simulink library "BFDAMP_MASTER"  (Simulink 8.5)
settings: Solver=ode45  StartTime=0.0  StopTime=10.0  RelTol=1e-3
libraries: cdsEpicsOut x36, cdsTP x18, cdsFiltCtrl x12, cdsFilt x12, cdsEpicsIn x7, cdsRms x6, cdsMuxMatrix x2, cdsEpicsBinIn x1, cdsFunctionCall x1, SIXOSEM_F_WD_AC_MASTER x1
(part 3 of 3)

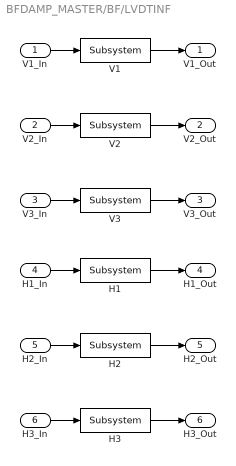
== system BFDAMP_MASTER/BF/LVDTINF ==
  V1_In : Inport
  V2_In : Inport  Port=2
  V3_In : Inport  Port=3
  H1_In : Inport  Port=4
  H2_In : Inport  Port=5
  H3_In : Inport  Port=6
  H1 : cdsFilt/Subsystem  Tag=cdsFilt  Description=|
      | Purpose:                                                                                                                                                                                                                                  
      | Standard CDS IIR filter module.                                                                                                                                                                                                           
      |                                                                                                                                                                                                                                           
      | Operation:                                                                                                                                                                                                                                
      | Consists of 10 second order section IIR filters, plus a ramped gain stage. In FE code, also provides pre-defined test points and excitation channel inputs. The filter coefficients are defined in the LIGO system using the 'foton' tool.
      |                                                                                                                                                                                                                                           
      | Usage:                                                                                                                                                                                                                                    
      | Name the part with the desired filter module name.
      settings: AttributesFormatString=%<Tag>
  H2 : cdsFilt/Subsystem  Tag=cdsFilt  Description=|
      | Purpose:                                                                                                                                                                                                                                  
      | Standard CDS IIR filter module.                                                                                                                                                                                                           
      |                                                                                                                                                                                                                                           
      | Operation:                                                                                                                                                                                                                                
      | Consists of 10 second order section IIR filters, plus a ramped gain stage. In FE code, also provides pre-defined test points and excitation channel inputs. The filter coefficients are defined in the LIGO system using the 'foton' tool.
      |                                                                                                                                                                                                                                           
      | Usage:                                                                                                                                                                                                                                    
      | Name the part with the desired filter module name.
      settings: AttributesFormatString=%<Tag>
  H3 : cdsFilt/Subsystem  Tag=cdsFilt  Description=|
      | Purpose:                                                                                                                                                                                                                                  
      | Standard CDS IIR filter module.                                                                                                                                                                                                           
      |                                                                                                                                                                                                                                           
      | Operation:                                                                                                                                                                                                                                
      | Consists of 10 second order section IIR filters, plus a ramped gain stage. In FE code, also provides pre-defined test points and excitation channel inputs. The filter coefficients are defined in the LIGO system using the 'foton' tool.
      |                                                                                                                                                                                                                                           
      | Usage:                                                                                                                                                                                                                                    
      | Name the part with the desired filter module name.
      settings: AttributesFormatString=%<Tag>
  V1 : cdsFilt/Subsystem  Tag=cdsFilt  Description=|
      | Purpose:                                                                                                                                                                                                                                  
      | Standard CDS IIR filter module.                                                                                                                                                                                                           
      |                                                                                                                                                                                                                                           
      | Operation:                                                                                                                                                                                                                                
      | Consists of 10 second order section IIR filters, plus a ramped gain stage. In FE code, also provides pre-defined test points and excitation channel inputs. The filter coefficients are defined in the LIGO system using the 'foton' tool.
      |                                                                                                                                                                                                                                           
      | Usage:                                                                                                                                                                                                                                    
      | Name the part with the desired filter module name.
      settings: AttributesFormatString=%<Tag>
  V2 : cdsFilt/Subsystem  Tag=cdsFilt  Description=|
      | Purpose:                                                                                                                                                                                                                                  
      | Standard CDS IIR filter module.                                                                                                                                                                                                           
      |                                                                                                                                                                                                                                           
      | Operation:                                                                                                                                                                                                                                
      | Consists of 10 second order section IIR filters, plus a ramped gain stage. In FE code, also provides pre-defined test points and excitation channel inputs. The filter coefficients are defined in the LIGO system using the 'foton' tool.
      |                                                                                                                                                                                                                                           
      | Usage:                                                                                                                                                                                                                                    
      | Name the part with the desired filter module name.
      settings: AttributesFormatString=%<Tag>
  V3 : cdsFilt/Subsystem  Tag=cdsFilt  Description=|
      | Purpose:                                                                                                                                                                                                                                  
      | Standard CDS IIR filter module.                                                                                                                                                                                                           
      |                                                                                                                                                                                                                                           
      | Operation:                                                                                                                                                                                                                                
      | Consists of 10 second order section IIR filters, plus a ramped gain stage. In FE code, also provides pre-defined test points and excitation channel inputs. The filter coefficients are defined in the LIGO system using the 'foton' tool.
      |                                                                                                                                                                                                                                           
      | Usage:                                                                                                                                                                                                                                    
      | Name the part with the desired filter module name.
      settings: AttributesFormatString=%<Tag>
  V1_Out : Outport
  V2_Out : Outport  Port=2
  V3_Out : Outport  Port=3
  H1_Out : Outport  Port=4
  H2_Out : Outport  Port=5
  H3_Out : Outport  Port=6
  wires:
  V1_In/1 -> V1/1
  V1/1 -> V1_Out/1
  V2_In/1 -> V2/1
  V2/1 -> V2_Out/1
  V3_In/1 -> V3/1
  V3/1 -> V3_Out/1
  H1_In/1 -> H1/1
  H1/1 -> H1_Out/1
  H2_In/1 -> H2/1
  H2/1 -> H2_Out/1
  H3_In/1 -> H3/1
  H3/1 -> H3_Out/1

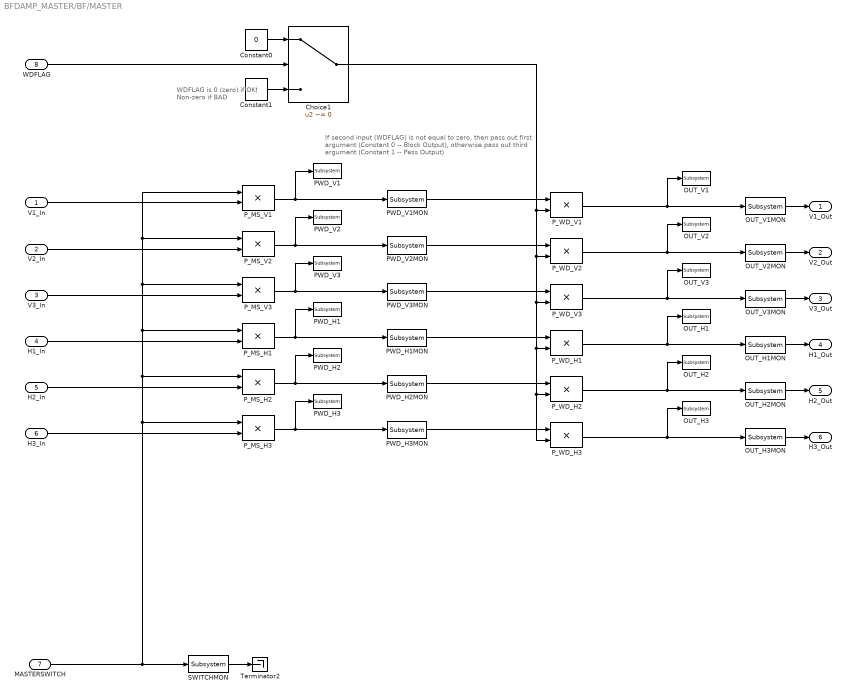
== system BFDAMP_MASTER/BF/MASTER ==
  note: If second input (WDFLAG) is not equal to zero,
      | then pass out first argument (Constant 0 -- Block Output),
      | otherwise pass out third argument (Constant 1 -- Pass Output)
  note: WDFLAG is 0 (zero) if OK,
      | Non-zero if BAD
  V1_In : Inport
  V2_In : Inport  Port=2
  V3_In : Inport  Port=3
  H1_In : Inport  Port=4
  H2_In : Inport  Port=5
  H3_In : Inport  Port=6
  MASTERSWITCH : Inport  Port=7
  WDFLAG : Inport  Port=8
  Choice1 : Switch  Criteria=u2 ~= 0  Threshold=0.5
  Constant0 : Constant  Value=0
  Constant1 : Constant
  OUT_H1 : cdsTP/Subsystem  Tag=Test Point
      settings: AttributesFormatString=%<Tag>
  OUT_H1MON : cdsEpicsOut/Subsystem  Tag=cdsEpicsOutput  Description=|
      | Purpose:                                          
      | Output a FE signal to an EPICS channel.           
      |                                                   
      | Operation:                                        
      | Takes input value and passes it to EPICS record.  
      |                                                   
      | Usage:                                            
      | Name the part with the desired EPICS rrecord name.
      settings: AttributesFormatString=%<Tag>
  OUT_H2 : cdsTP/Subsystem  Tag=Test Point
      settings: AttributesFormatString=%<Tag>
  OUT_H2MON : cdsEpicsOut/Subsystem  Tag=cdsEpicsOutput  Description=|
      | Purpose:                                          
      | Output a FE signal to an EPICS channel.           
      |                                                   
      | Operation:                                        
      | Takes input value and passes it to EPICS record.  
      |                                                   
      | Usage:                                            
      | Name the part with the desired EPICS rrecord name.
      settings: AttributesFormatString=%<Tag>
  OUT_H3 : cdsTP/Subsystem  Tag=Test Point
      settings: AttributesFormatString=%<Tag>
  OUT_H3MON : cdsEpicsOut/Subsystem  Tag=cdsEpicsOutput  Description=|
      | Purpose:                                          
      | Output a FE signal to an EPICS channel.           
      |                                                   
      | Operation:                                        
      | Takes input value and passes it to EPICS record.  
      |                                                   
      | Usage:                                            
      | Name the part with the desired EPICS rrecord name.
      settings: AttributesFormatString=%<Tag>
  OUT_V1 : cdsTP/Subsystem  Tag=Test Point
      settings: AttributesFormatString=%<Tag>
  OUT_V1MON : cdsEpicsOut/Subsystem  Tag=cdsEpicsOutput  Description=|
      | Purpose:                                          
      | Output a FE signal to an EPICS channel.           
      |                                                   
      | Operation:                                        
      | Takes input value and passes it to EPICS record.  
      |                                                   
      | Usage:                                            
      | Name the part with the desired EPICS rrecord name.
      settings: AttributesFormatString=%<Tag>
  OUT_V2 : cdsTP/Subsystem  Tag=Test Point
      settings: AttributesFormatString=%<Tag>
  OUT_V2MON : cdsEpicsOut/Subsystem  Tag=cdsEpicsOutput  Description=|
      | Purpose:                                          
      | Output a FE signal to an EPICS channel.           
      |                                                   
      | Operation:                                        
      | Takes input value and passes it to EPICS record.  
      |                                                   
      | Usage:                                            
      | Name the part with the desired EPICS rrecord name.
      settings: AttributesFormatString=%<Tag>
  OUT_V3 : cdsTP/Subsystem  Tag=Test Point
      settings: AttributesFormatString=%<Tag>
  OUT_V3MON : cdsEpicsOut/Subsystem  Tag=cdsEpicsOutput  Description=|
      | Purpose:                                          
      | Output a FE signal to an EPICS channel.           
      |                                                   
      | Operation:                                        
      | Takes input value and passes it to EPICS record.  
      |                                                   
      | Usage:                                            
      | Name the part with the desired EPICS rrecord name.
      settings: AttributesFormatString=%<Tag>
  PWD_H1 : cdsTP/Subsystem  Tag=Test Point
      settings: AttributesFormatString=%<Tag>
  PWD_H1MON : cdsEpicsOut/Subsystem  Tag=cdsEpicsOutput  Description=|
      | Purpose:                                          
      | Output a FE signal to an EPICS channel.           
      |                                                   
      | Operation:                                        
      | Takes input value and passes it to EPICS record.  
      |                                                   
      | Usage:                                            
      | Name the part with the desired EPICS rrecord name.
      settings: AttributesFormatString=%<Tag>
  PWD_H2 : cdsTP/Subsystem  Tag=Test Point
      settings: AttributesFormatString=%<Tag>
  PWD_H2MON : cdsEpicsOut/Subsystem  Tag=cdsEpicsOutput  Description=|
      | Purpose:                                          
      | Output a FE signal to an EPICS channel.           
      |                                                   
      | Operation:                                        
      | Takes input value and passes it to EPICS record.  
      |                                                   
      | Usage:                                            
      | Name the part with the desired EPICS rrecord name.
      settings: AttributesFormatString=%<Tag>
  PWD_H3 : cdsTP/Subsystem  Tag=Test Point
      settings: AttributesFormatString=%<Tag>
  PWD_H3MON : cdsEpicsOut/Subsystem  Tag=cdsEpicsOutput  Description=|
      | Purpose:                                          
      | Output a FE signal to an EPICS channel.           
      |                                                   
      | Operation:                                        
      | Takes input value and passes it to EPICS record.  
      |                                                   
      | Usage:                                            
      | Name the part with the desired EPICS rrecord name.
      settings: AttributesFormatString=%<Tag>
  PWD_V1 : cdsTP/Subsystem  Tag=Test Point
      settings: AttributesFormatString=%<Tag>
  PWD_V1MON : cdsEpicsOut/Subsystem  Tag=cdsEpicsOutput  Description=|
      | Purpose:                                          
      | Output a FE signal to an EPICS channel.           
      |                                                   
      | Operation:                                        
      | Takes input value and passes it to EPICS record.  
      |                                                   
      | Usage:                                            
      | Name the part with the desired EPICS rrecord name.
      settings: AttributesFormatString=%<Tag>
  PWD_V2 : cdsTP/Subsystem  Tag=Test Point
      settings: AttributesFormatString=%<Tag>
  PWD_V2MON : cdsEpicsOut/Subsystem  Tag=cdsEpicsOutput  Description=|
      | Purpose:                                          
      | Output a FE signal to an EPICS channel.           
      |                                                   
      | Operation:                                        
      | Takes input value and passes it to EPICS record.  
      |                                                   
      | Usage:                                            
      | Name the part with the desired EPICS rrecord name.
      settings: AttributesFormatString=%<Tag>
  PWD_V3 : cdsTP/Subsystem  Tag=Test Point
      settings: AttributesFormatString=%<Tag>
  PWD_V3MON : cdsEpicsOut/Subsystem  Tag=cdsEpicsOutput  Description=|
      | Purpose:                                          
      | Output a FE signal to an EPICS channel.           
      |                                                   
      | Operation:                                        
      | Takes input value and passes it to EPICS record.  
      |                                                   
      | Usage:                                            
      | Name the part with the desired EPICS rrecord name.
      settings: AttributesFormatString=%<Tag>
  P_MS_H1 : Product  RndMeth=Zero
  P_MS_H2 : Product  RndMeth=Zero
  P_MS_H3 : Product  RndMeth=Zero
  P_MS_V1 : Product  RndMeth=Zero
  P_MS_V2 : Product  RndMeth=Zero
  P_MS_V3 : Product  RndMeth=Zero
  P_WD_H1 : Product  RndMeth=Zero
  P_WD_H2 : Product  RndMeth=Zero
  P_WD_H3 : Product  RndMeth=Zero
  P_WD_V1 : Product  RndMeth=Zero
  P_WD_V2 : Product  RndMeth=Zero
  P_WD_V3 : Product  RndMeth=Zero
  SWITCHMON : cdsEpicsOut/Subsystem  Tag=cdsEpicsOutput  Description=|
      | Purpose:                                          
      | Output a FE signal to an EPICS channel.           
      |                                                   
      | Operation:                                        
      | Takes input value and passes it to EPICS record.  
      |                                                   
      | Usage:                                            
      | Name the part with the desired EPICS rrecord name.
      settings: AttributesFormatString=%<Tag>
  Terminator2 : Terminator
  V1_Out : Outport
  V2_Out : Outport  Port=2
  V3_Out : Outport  Port=3
  H1_Out : Outport  Port=4
  H2_Out : Outport  Port=5
  H3_Out : Outport  Port=6
  wires:
  SWITCHMON/1 -> Terminator2/1
  V1_In/1 -> P_MS_V1/2
  V2_In/1 -> P_MS_V2/2
  V3_In/1 -> P_MS_V3/2
  H1_In/1 -> P_MS_H1/2
  H2_In/1 -> P_MS_H2/2
  H3_In/1 -> P_MS_H3/2
  MASTERSWITCH/1 -> SWITCHMON/1, P_MS_V1/1, P_MS_V2/1, P_MS_V3/1, P_MS_H1/1, P_MS_H2/1, P_MS_H3/1
  OUT_V2MON/1 -> V2_Out/1
  OUT_V1MON/1 -> V1_Out/1
  OUT_V3MON/1 -> V3_Out/1
  OUT_H1MON/1 -> H1_Out/1
  OUT_H3MON/1 -> H3_Out/1
  OUT_H2MON/1 -> H2_Out/1
  P_MS_V1/1 -> PWD_V1/1, PWD_V1MON/1
  P_MS_V2/1 -> PWD_V2/1, PWD_V2MON/1
  P_MS_V3/1 -> PWD_V3/1, PWD_V3MON/1
  P_MS_H1/1 -> PWD_H1/1, PWD_H1MON/1
  P_MS_H2/1 -> PWD_H2/1, PWD_H2MON/1
  P_MS_H3/1 -> PWD_H3/1, PWD_H3MON/1
  P_WD_V1/1 -> OUT_V1MON/1, OUT_V1/1
  P_WD_V2/1 -> OUT_V2MON/1, OUT_V2/1
  P_WD_V3/1 -> OUT_V3MON/1, OUT_V3/1
  P_WD_H1/1 -> OUT_H1MON/1, OUT_H1/1
  P_WD_H2/1 -> OUT_H2MON/1, OUT_H2/1
  P_WD_H3/1 -> OUT_H3MON/1, OUT_H3/1
  Constant1/1 -> Choice1/3
  Constant0/1 -> Choice1/1
  WDFLAG/1 -> Choice1/2
  PWD_V1MON/1 -> P_WD_V1/1
  PWD_V2MON/1 -> P_WD_V2/1
  PWD_V3MON/1 -> P_WD_V3/1
  PWD_H1MON/1 -> P_WD_H1/1
  PWD_H2MON/1 -> P_WD_H2/1
  PWD_H3MON/1 -> P_WD_H3/1
  Choice1/1 -> P_WD_H3/2, P_WD_H2/2, P_WD_H1/2, P_WD_V3/2, P_WD_V2/2, P_WD_V1/2

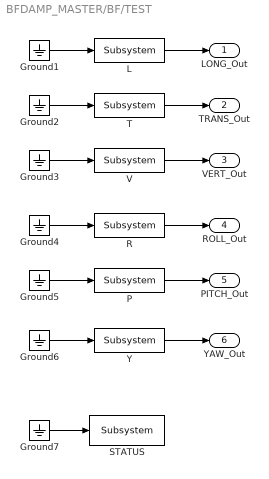
== system BFDAMP_MASTER/BF/TEST ==
  Ground{1..7} (7 alike) : Ground
  L : cdsFilt/Subsystem  Tag=cdsFilt  Description=|
      | Purpose:                                                                                                                                                                                                                                  
      | Standard CDS IIR filter module.                                                                                                                                                                                                           
      |                                                                                                                                                                                                                                           
      | Operation:                                                                                                                                                                                                                                
      | Consists of 10 second order section IIR filters, plus a ramped gain stage. In FE code, also provides pre-defined test points and excitation channel inputs. The filter coefficients are defined in the LIGO system using the 'foton' tool.
      |                                                                                                                                                                                                                                           
      | Usage:                                                                                                                                                                                                                                    
      | Name the part with the desired filter module name.
      settings: AttributesFormatString=%<Tag>
  P : cdsFilt/Subsystem  Tag=cdsFilt  Description=|
      | Purpose:                                                                                                                                                                                                                                  
      | Standard CDS IIR filter module.                                                                                                                                                                                                           
      |                                                                                                                                                                                                                                           
      | Operation:                                                                                                                                                                                                                                
      | Consists of 10 second order section IIR filters, plus a ramped gain stage. In FE code, also provides pre-defined test points and excitation channel inputs. The filter coefficients are defined in the LIGO system using the 'foton' tool.
      |                                                                                                                                                                                                                                           
      | Usage:                                                                                                                                                                                                                                    
      | Name the part with the desired filter module name.
      settings: AttributesFormatString=%<Tag>
  R : cdsFilt/Subsystem  Tag=cdsFilt  Description=|
      | Purpose:                                                                                                                                                                                                                                  
      | Standard CDS IIR filter module.                                                                                                                                                                                                           
      |                                                                                                                                                                                                                                           
      | Operation:                                                                                                                                                                                                                                
      | Consists of 10 second order section IIR filters, plus a ramped gain stage. In FE code, also provides pre-defined test points and excitation channel inputs. The filter coefficients are defined in the LIGO system using the 'foton' tool.
      |                                                                                                                                                                                                                                           
      | Usage:                                                                                                                                                                                                                                    
      | Name the part with the desired filter module name.
      settings: AttributesFormatString=%<Tag>
  STATUS : cdsEpicsBinIn/Subsystem  Tag=cdsEpicsBinIn  Description=|
      | Purpose:                                                                            
      | Create an EPICS binary (0 or 1) input channel to the FE realtime controls.          
      |                                                                                     
      | Operation:                                                                          
      | Outputs value from an EPICS ai record. Value is binary input (bi Epics record type).
      |                                                                                     
      | Usage:                                                                              
      | Name the part with the desired EPICS channel name.
      settings: AttributesFormatString=%<Tag>
  T : cdsFilt/Subsystem  Tag=cdsFilt  Description=|
      | Purpose:                                                                                                                                                                                                                                  
      | Standard CDS IIR filter module.                                                                                                                                                                                                           
      |                                                                                                                                                                                                                                           
      | Operation:                                                                                                                                                                                                                                
      | Consists of 10 second order section IIR filters, plus a ramped gain stage. In FE code, also provides pre-defined test points and excitation channel inputs. The filter coefficients are defined in the LIGO system using the 'foton' tool.
      |                                                                                                                                                                                                                                           
      | Usage:                                                                                                                                                                                                                                    
      | Name the part with the desired filter module name.
      settings: AttributesFormatString=%<Tag>
  V : cdsFilt/Subsystem  Tag=cdsFilt  Description=|
      | Purpose:                                                                                                                                                                                                                                  
      | Standard CDS IIR filter module.                                                                                                                                                                                                           
      |                                                                                                                                                                                                                                           
      | Operation:                                                                                                                                                                                                                                
      | Consists of 10 second order section IIR filters, plus a ramped gain stage. In FE code, also provides pre-defined test points and excitation channel inputs. The filter coefficients are defined in the LIGO system using the 'foton' tool.
      |                                                                                                                                                                                                                                           
      | Usage:                                                                                                                                                                                                                                    
      | Name the part with the desired filter module name.
      settings: AttributesFormatString=%<Tag>
  Y : cdsFilt/Subsystem  Tag=cdsFilt  Description=|
      | Purpose:                                                                                                                                                                                                                                  
      | Standard CDS IIR filter module.                                                                                                                                                                                                           
      |                                                                                                                                                                                                                                           
      | Operation:                                                                                                                                                                                                                                
      | Consists of 10 second order section IIR filters, plus a ramped gain stage. In FE code, also provides pre-defined test points and excitation channel inputs. The filter coefficients are defined in the LIGO system using the 'foton' tool.
      |                                                                                                                                                                                                                                           
      | Usage:                                                                                                                                                                                                                                    
      | Name the part with the desired filter module name.
      settings: AttributesFormatString=%<Tag>
  LONG_Out : Outport
  TRANS_Out : Outport  Port=2
  VERT_Out : Outport  Port=3
  ROLL_Out : Outport  Port=4
  PITCH_Out : Outport  Port=5
  YAW_Out : Outport  Port=6
  wires:
  Ground7/1 -> STATUS/1
  L/1 -> LONG_Out/1
  T/1 -> TRANS_Out/1
  V/1 -> VERT_Out/1
  Y/1 -> YAW_Out/1
  P/1 -> PITCH_Out/1
  R/1 -> ROLL_Out/1
  Ground1/1 -> L/1
  Ground2/1 -> T/1
  Ground3/1 -> V/1
  Ground6/1 -> Y/1
  Ground5/1 -> P/1
  Ground4/1 -> R/1

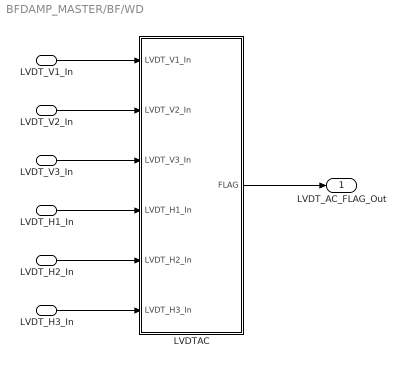
== system BFDAMP_MASTER/BF/WD ==
  LVDT_V1_In : Inport
  LVDT_V2_In : Inport  Port=2
  LVDT_V3_In : Inport  Port=3
  LVDT_H1_In : Inport  Port=4
  LVDT_H2_In : Inport  Port=5
  LVDT_H3_In : Inport  Port=6
  LVDTAC : Subsystem
  LVDT_AC_FLAG_Out : Outport
  wires:
  LVDT_V3_In/1 -> LVDTAC/3(LVDT_V3_In)
  LVDT_V2_In/1 -> LVDTAC/2(LVDT_V2_In)
  LVDT_V1_In/1 -> LVDTAC/1(LVDT_V1_In)
  LVDT_H1_In/1 -> LVDTAC/4(LVDT_H1_In)
  LVDT_H2_In/1 -> LVDTAC/5(LVDT_H2_In)
  LVDT_H3_In/1 -> LVDTAC/6(LVDT_H3_In)
  LVDTAC/1(FLAG) -> LVDT_AC_FLAG_Out/1

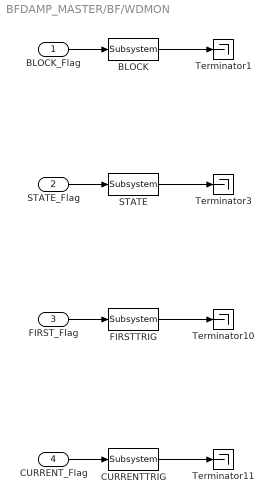
== system BFDAMP_MASTER/BF/WDMON ==
  BLOCK_Flag : Inport
  STATE_Flag : Inport  Port=2
  FIRST_Flag : Inport  Port=3
  CURRENT_Flag : Inport  Port=4
  BLOCK : cdsEpicsOut/Subsystem  Tag=cdsEpicsOutput  Description="field(PREC,\"3\")"
      settings: AttributesFormatString=%<Tag>
  CURRENTTRIG : cdsEpicsOut/Subsystem  Tag=cdsEpicsOutput  Description="field(PREC,\"3\")"
      settings: AttributesFormatString=%<Tag>
  FIRSTTRIG : cdsEpicsOut/Subsystem  Tag=cdsEpicsOutput  Description="field(PREC,\"3\")"
      settings: AttributesFormatString=%<Tag>
  STATE : cdsEpicsOut/Subsystem  Tag=cdsEpicsOutput  Description="field(PREC,\"3\")"
      settings: AttributesFormatString=%<Tag>
  Terminator{1,3,10..11} (4 alike) : Terminator
  wires:
  STATE/1 -> Terminator3/1
  BLOCK/1 -> Terminator1/1
  BLOCK_Flag/1 -> BLOCK/1
  FIRSTTRIG/1 -> Terminator10/1
  CURRENTTRIG/1 -> Terminator11/1
  CURRENT_Flag/1 -> CURRENTTRIG/1
  FIRST_Flag/1 -> FIRSTTRIG/1
  STATE_Flag/1 -> STATE/1

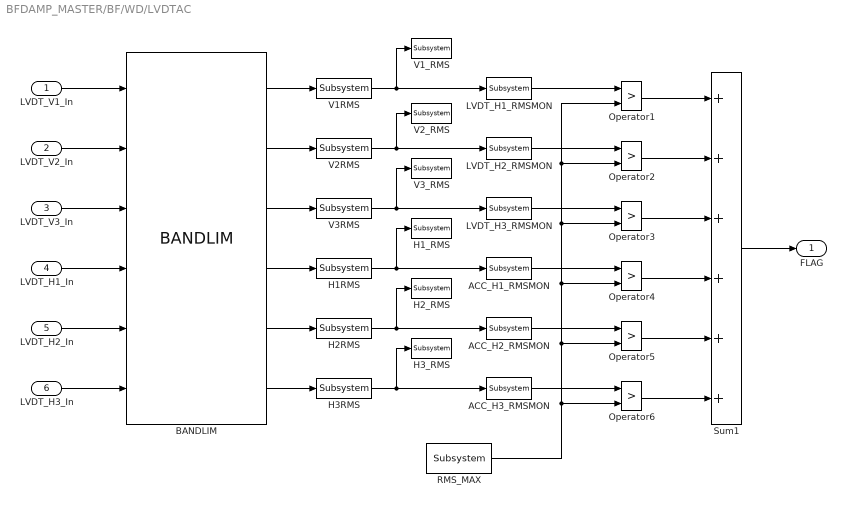
== system BFDAMP_MASTER/BF/WD/LVDTAC ==
  LVDT_V1_In : Inport
  LVDT_V2_In : Inport  Port=2
  LVDT_V3_In : Inport  Port=3
  LVDT_H1_In : Inport  Port=4
  LVDT_H2_In : Inport  Port=5
  LVDT_H3_In : Inport  Port=6
  ACC_H1_RMSMON : cdsEpicsOut/Subsystem  Tag=cdsEpicsOutput  Description=|
      | Purpose:                                          
      | Output a FE signal to an EPICS channel.           
      |                                                   
      | Operation:                                        
      | Takes input value and passes it to EPICS record.  
      |                                                   
      | Usage:                                            
      | Name the part with the desired EPICS rrecord name.
      settings: AttributesFormatString=%<Tag>
  ACC_H2_RMSMON : cdsEpicsOut/Subsystem  Tag=cdsEpicsOutput  Description=|
      | Purpose:                                          
      | Output a FE signal to an EPICS channel.           
      |                                                   
      | Operation:                                        
      | Takes input value and passes it to EPICS record.  
      |                                                   
      | Usage:                                            
      | Name the part with the desired EPICS rrecord name.
      settings: AttributesFormatString=%<Tag>
  ACC_H3_RMSMON : cdsEpicsOut/Subsystem  Tag=cdsEpicsOutput  Description=|
      | Purpose:                                          
      | Output a FE signal to an EPICS channel.           
      |                                                   
      | Operation:                                        
      | Takes input value and passes it to EPICS record.  
      |                                                   
      | Usage:                                            
      | Name the part with the desired EPICS rrecord name.
      settings: AttributesFormatString=%<Tag>
  BANDLIM : SIXOSEM_F_WD_AC_MASTER/AC/BANDLIM
  H1RMS : cdsRms/Subsystem  Tag=cdsRms  Description=|
      | Purpose:
      | Calculate an RMS based on the input signal.
      settings: AttributesFormatString=%<Tag>
  H1_RMS : cdsTP/Subsystem  Tag=Test Point
      settings: AttributesFormatString=%<Tag>
  H2RMS : cdsRms/Subsystem  Tag=cdsRms  Description=|
      | Purpose:
      | Calculate an RMS based on the input signal.
      settings: AttributesFormatString=%<Tag>
  H2_RMS : cdsTP/Subsystem  Tag=Test Point
      settings: AttributesFormatString=%<Tag>
  H3RMS : cdsRms/Subsystem  Tag=cdsRms  Description=|
      | Purpose:
      | Calculate an RMS based on the input signal.
      settings: AttributesFormatString=%<Tag>
  H3_RMS : cdsTP/Subsystem  Tag=Test Point
      settings: AttributesFormatString=%<Tag>
  LVDT_H1_RMSMON : cdsEpicsOut/Subsystem  Tag=cdsEpicsOutput  Description=|
      | Purpose:                                          
      | Output a FE signal to an EPICS channel.           
      |                                                   
      | Operation:                                        
      | Takes input value and passes it to EPICS record.  
      |                                                   
      | Usage:                                            
      | Name the part with the desired EPICS rrecord name.
      settings: AttributesFormatString=%<Tag>
  LVDT_H2_RMSMON : cdsEpicsOut/Subsystem  Tag=cdsEpicsOutput  Description=|
      | Purpose:                                          
      | Output a FE signal to an EPICS channel.           
      |                                                   
      | Operation:                                        
      | Takes input value and passes it to EPICS record.  
      |                                                   
      | Usage:                                            
      | Name the part with the desired EPICS rrecord name.
      settings: AttributesFormatString=%<Tag>
  LVDT_H3_RMSMON : cdsEpicsOut/Subsystem  Tag=cdsEpicsOutput  Description=|
      | Purpose:                                          
      | Output a FE signal to an EPICS channel.           
      |                                                   
      | Operation:                                        
      | Takes input value and passes it to EPICS record.  
      |                                                   
      | Usage:                                            
      | Name the part with the desired EPICS rrecord name.
      settings: AttributesFormatString=%<Tag>
  Operator{1,3..6} (5 alike) : RelationalOperator  Operator=>  OutDataTypeStr=boolean
  Operator2 : RelationalOperator  Operator=>  OutDataTypeStr=boolean  ZeroCross=off
  RMS_MAX : cdsEpicsIn/Subsystem  Tag=cdsEpicsIn  Description=|
      | Purpose:                                                                              
      | Create an EPICS input channel connection to the FE realtime controls.                 
      |                                                                                       
      | Operation:                                                                            
      | Outputs value from an EPICS ai record. Value is floating point with a precision of 3..
      |                                                                                       
      | Usage:                                                                                
      | Name the part with the desired EPICS channel name.
      settings: AttributesFormatString=%<Tag>
  Sum1 : Sum  Inputs=++++++
  V1RMS : cdsRms/Subsystem  Tag=cdsRms  Description=|
      | Purpose:
      | Calculate an RMS based on the input signal.
      settings: AttributesFormatString=%<Tag>
  V1_RMS : cdsTP/Subsystem  Tag=Test Point
      settings: AttributesFormatString=%<Tag>
  V2RMS : cdsRms/Subsystem  Tag=cdsRms  Description=|
      | Purpose:
      | Calculate an RMS based on the input signal.
      settings: AttributesFormatString=%<Tag>
  V2_RMS : cdsTP/Subsystem  Tag=Test Point
      settings: AttributesFormatString=%<Tag>
  V3RMS : cdsRms/Subsystem  Tag=cdsRms  Description=|
      | Purpose:
      | Calculate an RMS based on the input signal.
      settings: AttributesFormatString=%<Tag>
  V3_RMS : cdsTP/Subsystem  Tag=Test Point
      settings: AttributesFormatString=%<Tag>
  FLAG : Outport
  wires:
  BANDLIM/6 -> H3RMS/1
  BANDLIM/5 -> H2RMS/1
  BANDLIM/4 -> H1RMS/1
  BANDLIM/3 -> V3RMS/1
  BANDLIM/2 -> V2RMS/1
  BANDLIM/1 -> V1RMS/1
  LVDT_H3_In/1 -> BANDLIM/6
  LVDT_H2_In/1 -> BANDLIM/5
  LVDT_H1_In/1 -> BANDLIM/4
  LVDT_V3_In/1 -> BANDLIM/3
  LVDT_V2_In/1 -> BANDLIM/2
  LVDT_V1_In/1 -> BANDLIM/1
  Operator1/1 -> Sum1/1
  Operator2/1 -> Sum1/2
  Operator3/1 -> Sum1/3
  Operator4/1 -> Sum1/4
  RMS_MAX/1 -> Operator1/2, Operator2/2, Operator3/2, Operator4/2, Operator5/2, Operator6/2
  V2RMS/1 -> V2_RMS/1, LVDT_H2_RMSMON/1
  V1RMS/1 -> V1_RMS/1, LVDT_H1_RMSMON/1
  V3RMS/1 -> V3_RMS/1, LVDT_H3_RMSMON/1
  H1RMS/1 -> H1_RMS/1, ACC_H1_RMSMON/1
  Sum1/1 -> FLAG/1
  H2RMS/1 -> H2_RMS/1, ACC_H2_RMSMON/1
  H3RMS/1 -> H3_RMS/1, ACC_H3_RMSMON/1
  LVDT_H1_RMSMON/1 -> Operator1/1
  LVDT_H2_RMSMON/1 -> Operator2/1
  LVDT_H3_RMSMON/1 -> Operator3/1
  ACC_H1_RMSMON/1 -> Operator4/1
  ACC_H2_RMSMON/1 -> Operator5/1
  ACC_H3_RMSMON/1 -> Operator6/1
  Operator5/1 -> Sum1/5
  Operator6/1 -> Sum1/6
